simulink model "Improved_Final_Model"  (R2022a)
settings: Solver=FixedStepAuto  StartTime=0.0  StopTime=10.0  FixedStep=1e-3  RelTol=1e-3  EnableMultiTasking=on
undefined symbols (not defined in the file): a, A0, A1, b, c, D0, D1, D10, D11, D12, D13, D2, D3, D5, D6, D8, D9, PTA0, PTA1, PTA2, PTB2, PTB3, PTB9, PTC16, PTC17, PTC2, PTC4, PTD0, PTD1, PTD2, PTD3
libraries: frdmk64flib x17, simulink x2, hdlsllib x1
settings Model: ExtModeTrigDuration=5  Creator=pauls  LastModifiedBy=pauls
settings OptimizationCC: EnhancedBackFolding=on  PassReuseOutputArgsAs=Individual arguments  ZeroExternalMemoryAtStartup=off  ZeroInternalMemoryAtStartup=off  MaxStackSize=64  OptimizeBlockOrder=speed  DifferentSizesBufferReuse=on  OptimizationCustomize=off  EfficientTunableParamExpr=on
settings DebuggingCC: ParameterTunabilityLossMsg=error
settings HardwareCC: ProdBitPerPointer=32  ProdBitPerSizeT=32  ProdBitPerPtrDiffT=32  ProdLargestAtomicInteger=Long  ProdLargestAtomicFloat=Double  ProdWordSize=32  ProdHWDeviceType=ARM Compatible->ARM Cortex
settings SFSimCC: MATLABDynamicMemAlloc=off
settings RTWCC: SystemTargetFile=ert.tlc  HardwareBoard=NXP FRDM-K64F  TLCOptions="-aInlineSetEventsForThisBaseRateFcn=TLC_FALSE -aSuppressMultiTaskScheduler=TLC_FALSE  -aRateBasedStepFcn=0"  TemplateMakefile=ert_default_tmf  Toolchain=GNU Tools for ARM Embedded Processors
settings CodeAppCC: ForceParamTrailComments=on  IgnoreCustomStorageClasses=off  OperatorAnnotations=on  SimulinkDataObjDesc=on  SFDataObjDesc=on  InsertBlockDesc=on
settings ERTTargetCC: ExtModeTransport=4  ExtModeMexFile=sendToCommService

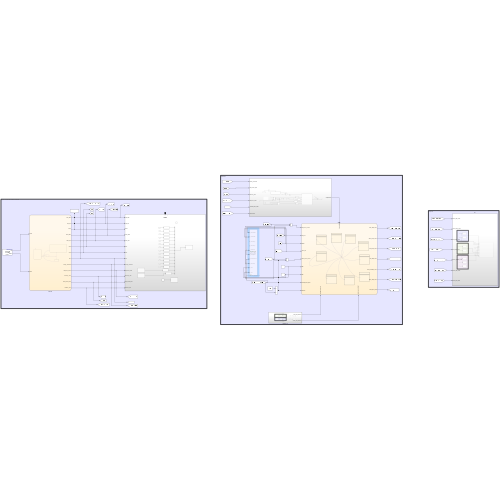
[thumbnail: Simulink's stored preview of the top-level diagram]
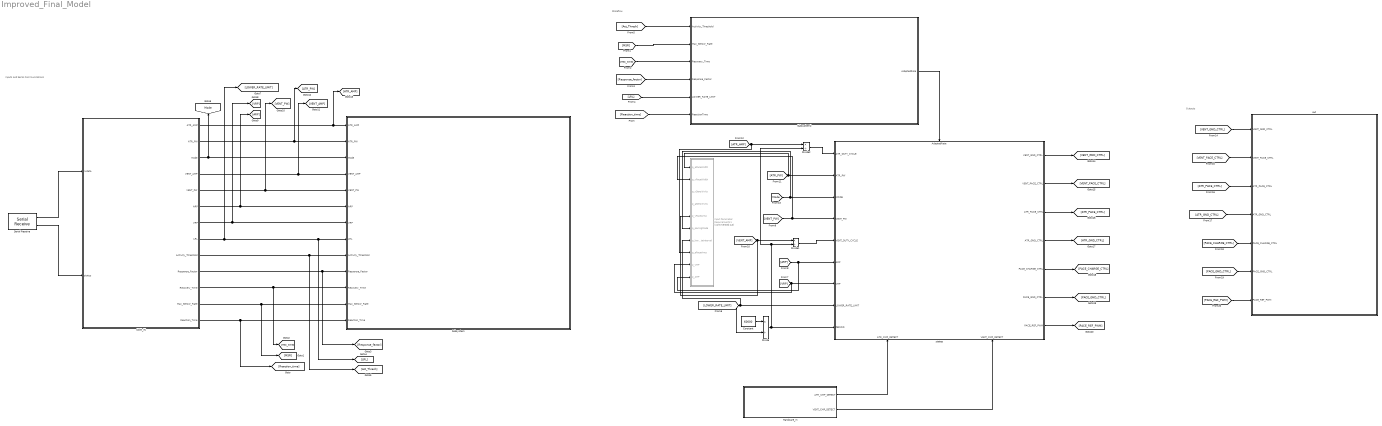
== system Improved_Final_Model ==
  note: Outputs
  note: Stateflow
  note: Inputs and Serial Communications
  " states  " : Stateflow chart  TreatAsAtomicUnit=on
      settings: PortSchema="{\"entries\":[{\"content\":{\"sides\":[{\"content\":{\"connectorIds\":[\"In7\",\"In8\",\"In2\",\"In5\",\"In6\",\"In11\",\"In10\",\"In12\",\"In9\"]},\"type\":\"ConnectorPlacement.EquallySpacedRectSide\",\"uuid\":\"01118a3a-35ab-415d-a4dc-7a9e5022dc58\"},{\"content\":{\"connectorIds\":[\"Out1\",\"Out2\",\"Out3\",\"Out4\",\"Out5\",\"Out6\",\"Out7\"],\"side\":\"RIGHT\"},\"type\":\"ConnectorPlacement.EquallySpacedRectSide\",\"uuid\":\"d119b6db-c579-45b6-8580-2a3960ab3129\"},{\"content\":{\"connectorIds\":[\"In1\"],\"side\":\"TOP\"},\"type\":\"ConnectorPlacement.EquallySpacedRectSide\",\"uuid\":\"18fa5379-1691-4053-811b-8d647a346445\"},{\"content\":{\"connectorIds\":[\"In3\",\"In4\"],\"side\":\"BOTTOM\"},\"type\":\"ConnectorPlacement.EquallySpacedRectSide\",\"uuid\":\"c19ca9f7-b829-4e11-b03e-3e9d42b35795\"}]},\"type\":\"ConnectorPlacement.EquallySpacedConnector\",\"uuid\":\"6e6fa963-33ea-4c14-97b4-73e5587667a9\"}],\"packageUris\":[\"http://schema.mathworks.com/mf0/Connector/R2020b\"],\"version\":\"1.0\"}"
  COM_IN : Stateflow chart  TreatAsAtomicUnit=on
      settings: PortSchema="{\"entries\":[{\"content\":{\"sides\":[{\"content\":{\"connectorIds\":[\"In1\",\"In2\"]},\"type\":\"ConnectorPlacement.EquallySpacedRectSide\",\"uuid\":\"47dbc3b1-cfb0-4419-87af-22cc7bee4e7f\"},{\"content\":{\"connectorIds\":[\"Out2\",\"Out1\",\"Out3\",\"Out4\",\"Out5\",\"Out6\",\"Out7\",\"Out8\",\"Out9\",\"Out10\",\"Out11\",\"Out12\",\"Out13\"],\"side\":\"RIGHT\"},\"type\":\"ConnectorPlacement.EquallySpacedRectSide\",\"uuid\":\"7e5976fa-7974-49bc-a061-2d3361778a3d\"},{\"content\":{\"connectorIds\":[],\"side\":\"TOP\"},\"type\":\"ConnectorPlacement.EquallySpacedRectSide\",\"uuid\":\"f4969c99-fcc1-4334-9f12-327b19c61b40\"}]},\"type\":\"ConnectorPlacement.EquallySpacedConnector\",\"uuid\":\"ac43404f-f257-440c-be82-ec9e7dd20d0c\"}],\"packageUris\":[\"http://schema.mathworks.com/mf0/Connector/R2020b\"],\"version\":\"1.0\"}"
  Constant : Constant  Value=60000
  Divide : Product  Inputs=*/
  Divide1 : Product  Inputs=*/
  Divide2 : Product  Inputs=*/
  Hardware_in : Subsystem
  Input Parameter Requirements1 : Requirements Table  Commented=on  TreatAsAtomicUnit=on
  Serial Receive : frdmk64flib/Serial Receive  SCIModule=0  Baudrate=uint32(9600)  Parity=None  StopBits=1  HardwareFlowControl=None  ByteOrder=LittleEndian  DataType=uint8  DataLength=15  BlockingMode=off  OutputStatus=on  SampleTime=-1
  Subsystem : Subsystem
  Subsystem2 : Subsystem
  "out " : Subsystem
  tag scope: Mode=global
  wires:
  Serial Receive/1 -> COM_IN/1(rxdata)
  Serial Receive/2 -> COM_IN/2(status)
  COM_IN/1(ATR_PW) -> [ATR_PW], Subsystem/2(ATR_PW)
  COM_IN/2(ATR_AMP) -> [ATR_AMP], Subsystem/1(ATR_AMP)
  COM_IN/3(Mode) -> Subsystem/3(Mode), [Mode]
  COM_IN/4(VENT_AMP) -> [VENT_AMP], Subsystem/4(VENT_AMP)
  COM_IN/5(VENT_PW) -> [VENT_PW], Subsystem/5(VENT_PW)
  COM_IN/6(ARP) -> [ARP], Subsystem/6(ARP)
  COM_IN/7(VRP) -> [VRP], Subsystem/7(VRP)
  COM_IN/8(LRL) -> [LOWER_RATE_LIMIT], [LRL], Subsystem/8(LRL)
  COM_IN/9(Activity_Threshold) -> [Act_Thresh], Subsystem/9(Activity_Threshold)
  COM_IN/10(Response_Factor) -> [Response_factor], Subsystem/10(Response_Factor)
  COM_IN/11(Recovery_Time) -> [Rec_time], Subsystem/11(Recovery_Time)
  COM_IN/12(Max_Sensor_Rate) -> [MSR], Subsystem/12(Max_Sensor_Rate)
  COM_IN/13(Reaction_Time) -> Subsystem/13(Reaction_Time), [Reaction_time]
  Hardware_in/1(ATR_CMP_DETECT) -> " states  "/3(ATR_CMP_DETECT)
  Hardware_in/2(VENT_CMP_DETECT) -> " states  "/4(VENT_CMP_DETECT)
  Divide/1 -> Divide1/2, Divide2/2, " states  "/9(PERIOD)
  Constant/1 -> Divide/1
  [Rec_time] -> Subsystem2/3(Recovery_Time)
  [Response_factor] -> Subsystem2/4(Response_Factor)
  [LRL] -> Subsystem2/5(LOWER_RATE_LIMIT)
  [Reaction_time] -> Subsystem2/6(ReactionTime)
  [Act_Thresh] -> Subsystem2/1(Activity_Threshold)
  [MSR] -> Subsystem2/2(Max_Sensor_Rate)
  Subsystem2/1(AdaptedRate) -> " states  "/1(AdaptedRate)
  [LOWER_RATE_LIMIT] -> Input Parameter Requirements1/7(p_lowrateInterval), " states  "/12(LOWER_RATE_LIMIT), Divide/2
  [VRP] -> Input Parameter Requirements1/9(p_VRP), " states  "/10(VRP)
  [ARP] -> Input Parameter Requirements1/10(p_ARP), " states  "/11(ARP)
  [ATR_PW] -> Input Parameter Requirements1/1(p_aPaceWidth), " states  "/8(ATR_PW)
  [VENT_AMP] -> Input Parameter Requirements1/5(p_vPaceAmp), Divide1/1
  [VENT_PW] -> Input Parameter Requirements1/2(p_vPaceWidth), " states  "/5(VENT_PW)
  [ATR_AMP] -> Input Parameter Requirements1/8(p_aPaceAmp), Divide2/1
  [Mode] -> Input Parameter Requirements1/6(p_pacingMode), " states  "/2(MODE)
  " states  "/1(VENT_GND_CTRL) -> [VENT_GND_CTRL]
  " states  "/2(VENT_PACE_CTRL) -> [VENT_PACE_CTRL]
  " states  "/3(ATR_PACE_CTRL) -> [ATR_PACE_CTRL]
  " states  "/4(ATR_GND_CTRL) -> [ATR_GND_CTRL]
  " states  "/5(PACE_CHARGE_CTRL) -> [PACE_CHARGE_CTRL]
  " states  "/6(PACE_GND_CTRL) -> [PACE_GND_CTRL]
  " states  "/7(PACE_REF_PWM) -> [PACE_REF_PWM]
  [VENT_GND_CTRL] -> "out "/1(VENT_GND_CTRL)
  [VENT_PACE_CTRL] -> "out "/2(VENT_PACE_CTRL)
  [ATR_PACE_CTRL] -> "out "/3(ATR_PACE_CTRL)
  [ATR_GND_CTRL] -> "out "/4(ATR_GND_CTRL)
  [PACE_CHARGE_CTRL] -> "out "/5(PACE_CHARGE_CTRL)
  [PACE_GND_CTRL] -> "out "/6(PACE_GND_CTRL)
  [PACE_REF_PWM] -> "out "/7(PACE_REF_PWM)
  Divide1/1 -> " states  "/6(VENT_DUTY_CYCLE)
  Divide2/1 -> " states  "/7(ATR_DUTY_CYCLE)

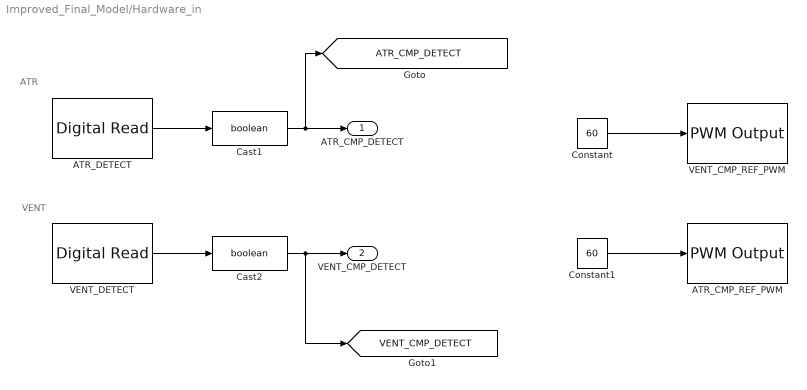
== system Improved_Final_Model/Hardware_in ==
  note: VENT
  note: ATR
  ATR_CMP_REF_PWM : frdmk64flib/PWM Output  Whichpin=PTC2 (D6)  InitialFrequency=2000  InitialDutyCycle=52
  ATR_DETECT : frdmk64flib/Digital Read  Whichpin=PTC16 (D0)  SampleTime=-1
  Cast1 : DataTypeConversion  OutDataTypeStr=boolean  SaturateOnIntegerOverflow=off  RndMeth=Floor
  Cast2 : DataTypeConversion  OutDataTypeStr=boolean  SaturateOnIntegerOverflow=off  RndMeth=Floor
  Constant : Constant  Value=60
  Constant1 : Constant  Value=60
  VENT_CMP_REF_PWM : frdmk64flib/PWM Output  Whichpin=PTA1 (D3)  InitialFrequency=2000  InitialDutyCycle=52
  VENT_DETECT : frdmk64flib/Digital Read  Whichpin=PTC17 (D1)  SampleTime=-1
  ATR_CMP_DETECT : Outport
  VENT_CMP_DETECT : Outport  Port=2
  tag scope: ATR_CMP_DETECT=global, VENT_CMP_DETECT=global
  wires:
  Cast1/1 -> ATR_CMP_DETECT/1, [ATR_CMP_DETECT]
  ATR_DETECT/1 -> Cast1/1
  VENT_DETECT/1 -> Cast2/1
  Cast2/1 -> [VENT_CMP_DETECT], VENT_CMP_DETECT/1
  Constant/1 -> VENT_CMP_REF_PWM/1
  Constant1/1 -> ATR_CMP_REF_PWM/1

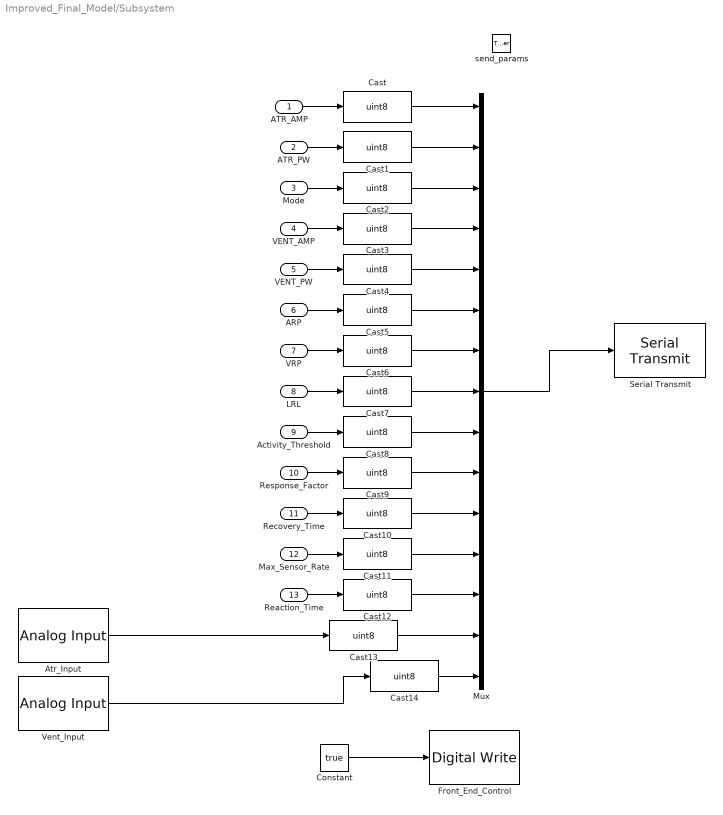
== system Improved_Final_Model/Subsystem ==
  ATR_AMP : Inport
  ATR_PW : Inport  Port=2
  Mode : Inport  Port=3
  VENT_AMP : Inport  Port=4
  VENT_PW : Inport  Port=5
  ARP : Inport  Port=6
  VRP : Inport  Port=7
  LRL : Inport  Port=8
  Activity_Threshold : Inport  Port=9
  Response_Factor : Inport  Port=10
  Recovery_Time : Inport  Port=11
  Max_Sensor_Rate : Inport  Port=12
  Reaction_Time : Inport  Port=13
  send_params : TriggerPort  TriggerType=function-call  IsSimulinkFunction=on  FunctionName=send_Test  VariantControl=(inherit)
  Atr_Input : frdmk64flib/Analog Input  Whichpin=PTB2 (A0)  SampleTime=-1
  Cast{,1..14} (15 alike) : DataTypeConversion  OutDataTypeStr=uint8  SaturateOnIntegerOverflow=off  RndMeth=Floor
  Constant : Constant  Value=true
  Front_End_Control : frdmk64flib/Digital Write  Whichpin=PTD1 (D13)
  Mux : Mux  Inputs=15
  Serial Transmit : frdmk64flib/Serial Transmit  SCIModule=0  Baudrate=uint32(9600)  Parity=None  StopBits=1  HardwareFlowControl=None  ByteOrder=LittleEndian  BlockingMode=on  OutputStatus=off
  Vent_Input : frdmk64flib/Analog Input  Whichpin=PTB3 (A1)  SampleTime=-1
  wires:
  ATR_AMP/1 -> Cast/1
  Mux/1 -> Serial Transmit/1
  ATR_PW/1 -> Cast1/1
  Cast1/1 -> Mux/2
  Cast/1 -> Mux/1
  Mode/1 -> Cast2/1
  Cast2/1 -> Mux/3
  VENT_AMP/1 -> Cast3/1
  VENT_PW/1 -> Cast4/1
  ARP/1 -> Cast5/1
  VRP/1 -> Cast6/1
  LRL/1 -> Cast7/1
  Cast3/1 -> Mux/4
  Cast4/1 -> Mux/5
  Cast5/1 -> Mux/6
  Cast6/1 -> Mux/7
  Cast7/1 -> Mux/8
  Cast8/1 -> Mux/9
  Cast12/1 -> Mux/13
  Cast11/1 -> Mux/12
  Cast9/1 -> Mux/10
  Cast10/1 -> Mux/11
  Response_Factor/1 -> Cast9/1
  Activity_Threshold/1 -> Cast8/1
  Recovery_Time/1 -> Cast10/1
  Reaction_Time/1 -> Cast12/1
  Max_Sensor_Rate/1 -> Cast11/1
  Constant/1 -> Front_End_Control/1
  Atr_Input/1 -> Cast13/1
  Vent_Input/1 -> Cast14/1
  Cast13/1 -> Mux/14
  Cast14/1 -> Mux/15

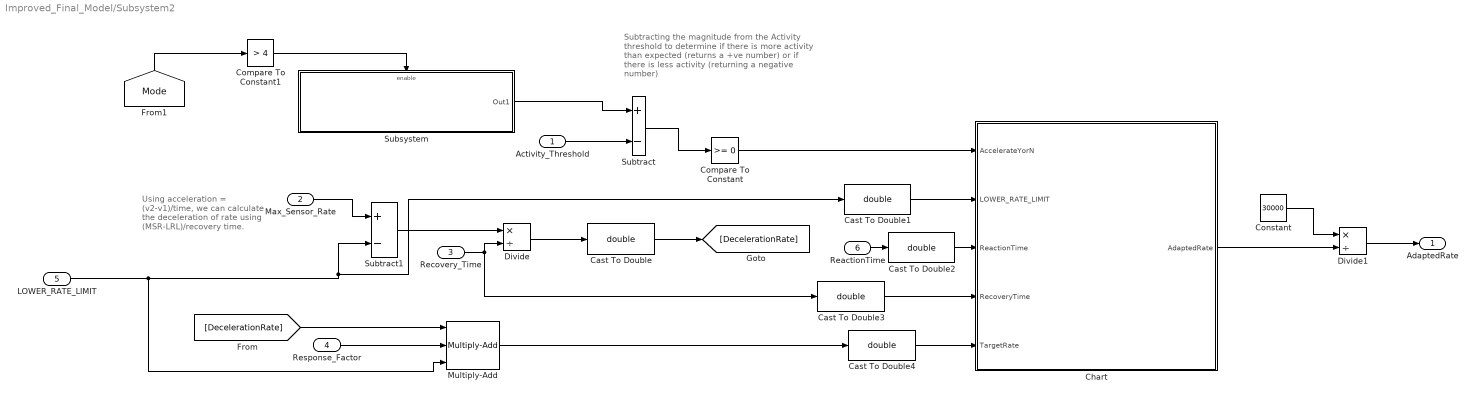
== system Improved_Final_Model/Subsystem2 ==
  note: Using acceleration = (v2-v1)/time, we can calculate the deceleration of rate using
      | (MSR-LRL)/recovery time.
  note: Subtracting the magnitude from the Activity threshold to determine if there is more activity than expected (returns a +ve number) or if there is less activity (returning a negative number)
  Activity_Threshold : Inport
  Max_Sensor_Rate : Inport  Port=2
  Recovery_Time : Inport  Port=3
  Response_Factor : Inport  Port=4
  LOWER_RATE_LIMIT : Inport  Port=5
  ReactionTime : Inport  Port=6
  Cast To Double{,1..4} (5 alike) : DataTypeConversion  OutDataTypeStr=double  SaturateOnIntegerOverflow=off  RndMeth=Floor
  Chart : Stateflow chart  TreatAsAtomicUnit=on
      settings: PortSchema="{\"entries\":[{\"content\":{\"sides\":[{\"content\":{\"connectorIds\":[\"In2\",\"In1\",\"In3\",\"In4\",\"In5\"]},\"type\":\"ConnectorPlacement.EquallySpacedRectSide\",\"uuid\":\"6eaaa5c3-a67e-4334-8771-4d714dd3c2aa\"},{\"content\":{\"connectorIds\":[\"Out1\"],\"side\":\"RIGHT\"},\"type\":\"ConnectorPlacement.EquallySpacedRectSide\",\"uuid\":\"be5e1652-7b89-433f-97fe-a51584ee4ad6\"},{\"content\":{\"connectorIds\":[],\"side\":\"TOP\"},\"type\":\"ConnectorPlacement.EquallySpacedRectSide\",\"uuid\":\"88923a53-eca7-4a95-abe6-229d007878e0\"}]},\"type\":\"ConnectorPlacement.EquallySpacedConnector\",\"uuid\":\"0db105c6-87da-444f-9a1d-26abcd68563f\"}],\"packageUris\":[\"http://schema.mathworks.com/mf0/Connector/R2020b\"],\"version\":\"1.0\"}"
  Compare To Constant : simulink/Logic and Bit Operations/Compare To Constant  relop=>=  const=0  OutDataTypeStr=boolean
  Compare To Constant1 : simulink/Logic and Bit Operations/Compare To Constant  relop=>  const=4  OutDataTypeStr=boolean
  Constant : Constant  Value=30000
  Divide : Product  Inputs=*/
  Divide1 : Product  Inputs=*/
  Multiply-Add : hdlsllib/HDL Operations/Multiply-Add  Function=c+(a.*b)  datatype=Inherit: Inherit via internal rule  DoSatur=off  FMA=off
      settings: SourceProductBaseCode=SL
  Subsystem : Subsystem
  Subtract : Sum  Inputs=+-
  Subtract1 : Sum  Inputs=+-
  AdaptedRate : Outport
  wires:
  Divide1/1 -> AdaptedRate/1
  Response_Factor/1 -> Multiply-Add/2
  Cast To Double2/1 -> Chart/3(ReactionTime)
  Cast To Double4/1 -> Chart/5(TargetRate)
  ReactionTime/1 -> Cast To Double2/1
  Cast To Double1/1 -> Chart/1(LOWER_RATE_LIMIT)
  [DecelerationRate] -> Multiply-Add/1
  Constant/1 -> Divide1/1
  Subtract1/1 -> Divide/1
  Cast To Double3/1 -> Chart/4(RecoveryTime)
  Chart/1(AdaptedRate) -> Divide1/2
  Recovery_Time/1 -> Cast To Double3/1, Divide/2
  LOWER_RATE_LIMIT/1 -> Multiply-Add/3, Subtract1/2, Cast To Double1/1
  Cast To Double/1 -> [DecelerationRate]
  Compare To Constant/1 -> Chart/2(AccelerateYorN)
  Divide/1 -> Cast To Double/1
  Max_Sensor_Rate/1 -> Subtract1/1
  Activity_Threshold/1 -> Subtract/2
  Subtract/1 -> Compare To Constant/1
  Multiply-Add/1 -> Cast To Double4/1
  Subsystem/1(Out1) -> Subtract/1
  [Mode] -> Compare To Constant1/1
  Compare To Constant1/1 -> Subsystem/Enable

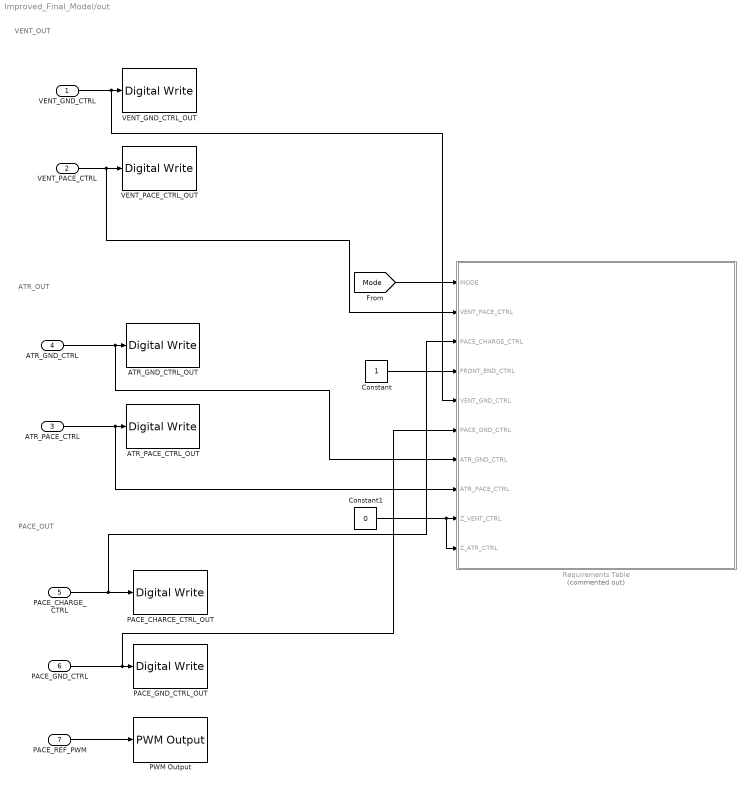
== system Improved_Final_Model/out  ==
  note: PACE_OUT
  note: ATR_OUT
  note: VENT_OUT
  VENT_GND_CTRL : Inport
  VENT_PACE_CTRL : Inport  Port=2
  ATR_PACE_CTRL : Inport  Port=3
  ATR_GND_CTRL : Inport  Port=4
  PACE_CHARGE_CTRL : Inport  Port=5
  PACE_GND_CTRL : Inport  Port=6
  PACE_REF_PWM : Inport  Port=7
  ATR_GND_CTRL_OUT : frdmk64flib/Digital Write  Whichpin=PTD2 (D11)
  ATR_PACE_CTRL_OUT : frdmk64flib/Digital Write  Whichpin=PTA0 (D8)
  Constant : Constant
  Constant1 : Constant  Value=0
  PACE_CHARCE_CTRL_OUT : frdmk64flib/Digital Write  Whichpin=PTB9 (D2)
  PACE_GND_CTRL_OUT : frdmk64flib/Digital Write  Whichpin=PTD0 (D10)
  PWM Output : frdmk64flib/PWM Output  Whichpin=PTA2 (D5)  InitialFrequency=2000  InitialDutyCycle=100
  Requirements Table : Requirements Table  Commented=on  TreatAsAtomicUnit=on
  VENT_GND_CTRL_OUT : frdmk64flib/Digital Write  Whichpin=PTD3 (D12)
  VENT_PACE_CTRL_OUT : frdmk64flib/Digital Write  Whichpin=PTC4 (D9)
  wires:
  VENT_GND_CTRL/1 -> Requirements Table/5(VENT_GND_CTRL), VENT_GND_CTRL_OUT/1
  VENT_PACE_CTRL/1 -> Requirements Table/2(VENT_PACE_CTRL), VENT_PACE_CTRL_OUT/1
  ATR_GND_CTRL/1 -> Requirements Table/7(ATR_GND_CTRL), ATR_GND_CTRL_OUT/1
  ATR_PACE_CTRL/1 -> Requirements Table/8(ATR_PACE_CTRL), ATR_PACE_CTRL_OUT/1
  PACE_CHARGE_CTRL/1 -> Requirements Table/3(PACE_CHARGE_CTRL), PACE_CHARCE_CTRL_OUT/1
  PACE_REF_PWM/1 -> PWM Output/1
  PACE_GND_CTRL/1 -> Requirements Table/6(PACE_GND_CTRL), PACE_GND_CTRL_OUT/1
  [Mode] -> Requirements Table/1(MODE)
  Constant/1 -> Requirements Table/4(FRONT_END_CTRL)
  Constant1/1 -> Requirements Table/10(Z_ATR_CTRL), Requirements Table/9(Z_VENT_CTRL)

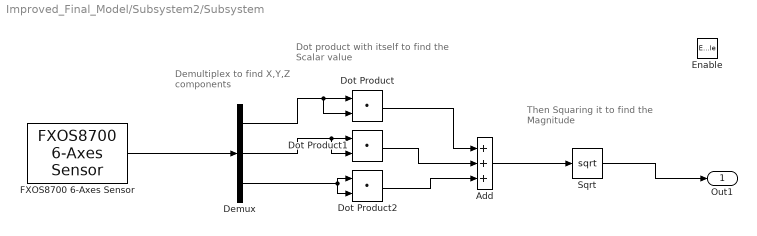
== system Improved_Final_Model/Subsystem2/Subsystem ==
  note: Demultiplex to find
      | X,Y,Z components
  note: Dot product with itself to find the
      | Scalar value
  note: Then Squaring it to find the Magnitude
  Enable : EnablePort
  Add : Sum  Inputs=+++
  Demux : Demux  Outputs=3
  Dot Product : DotProduct  OutDataTypeStr=Inherit: Inherit via internal rule
  Dot Product1 : DotProduct  OutDataTypeStr=Inherit: Inherit via internal rule
  Dot Product2 : DotProduct  OutDataTypeStr=Inherit: Inherit via internal rule
  FXOS8700 6-Axes Sensor : frdmk64flib/FXOS8700 6-Axes Sensor  Activesensor=Accelerometer only  ODR=800Hz  HybridODR=400Hz  Accelfullrange=-4g to +4g  SampleTime=-1
  Sqrt : Sqrt
  Out1 : Outport
  wires:
  Demux/3 -> Dot Product2/2, Dot Product2/1
  Demux/2 -> Dot Product1/2, Dot Product1/1
  Demux/1 -> Dot Product/2, Dot Product/1
  FXOS8700 6-Axes Sensor/1 -> Demux/1
  Dot Product2/1 -> Add/3
  Dot Product/1 -> Add/1
  Add/1 -> Sqrt/1
  Dot Product1/1 -> Add/2
  Sqrt/1 -> Out1/1

== stateflow chart Improved_Final_Model/ states   ==
  state Default [group]
    state CharingC23
      during:
      %Begin Charging C22 Capacitor
      VENT_PACE_CTRL = LOW;
      PACE_REF_PWM = (VENT_DUTY_CYCLE/5)*100;
      PACE_CHARGE_CTRL = HIGH;
      %Begin Discharging C21 Blocking Capacitor
      PACE_GND_CTRL = HIGH;
      VENT_PACE_CTRL = LOW;
      VENT_GND_CTRL = HIGH;
    state Discharge
      during:
      %Discharge C22 into Ventricle (Vent Pacing)
      %Begin Charging Blocking Capacitor
      PACE_CHARGE_CTRL = LOW;
      PACE_GND_CTRL = HIGH;
      VENT_GND_CTRL = LOW;
      VENT_PACE_CTRL  = HIGH;
    Default.CharingC23 -> Default.Discharge : after(PERIOD-VENT_PW, msec)
    Default.Discharge -> Default.CharingC23 : after(VENT_PW, msec)
  state AOO [group]
    state CharingC22
      %Capacitor charing state
      ATR_PACE_CTRL = LOW
      PACE_REF_PWM = (ATR_DUTY_CYCLE/5)*100
      PACE_CHARGE_CTRL = HIGH
      %Discharge capacitor
      PACE_GND_CTRL = HIGH
      ATR_PACE_CTRL = LOW
      ATR_GND_CTRL = HIGH
    state AVPacing
      %step 2
      PACE_CHARGE_CTRL = LOW
      PACE_GND_CTRL = HIGH
      ATR_PACE_CTRL = HIGH
      ATR_GND_CTRL = LOW
    AOO.CharingC22 -> AOO.AVPacing : after(PERIOD-ATR_PW, msec)
    AOO.AVPacing -> AOO.CharingC22 : after(ATR_PW, msec)
  state VVIR [group]
    state DISCHARGING
      during:
      %Step 1:
      %Discharge C22 into Ventricle (Vent Pacing)
      %Begin Charging Blocking Capacitor
      PACE_CHARGE_CTRL = LOW
      PACE_GND_CTRL = HIGH
      VENT_GND_CTRL = LOW
      VENT_PACE_CTRL  = HIGH
    state CHARGING
      during:
      %Begin Charging C22 Capacitor
      VENT_PACE_CTRL = LOW;
      PACE_REF_PWM = (VENT_DUTY_CYCLE/5)*100;
      PACE_CHARGE_CTRL = HIGH;
      %Begin Discharging C21 Blocking Capacitor
      PACE_GND_CTRL = HIGH;
      VENT_PACE_CTRL = LOW;
      VENT_GND_CTRL = HIGH;
    state PROXY
      during:
      PACE_GND_CTRL = HIGH;
      VENT_PACE_CTRL = LOW;
      VENT_GND_CTRL = HIGH;
    CHARGING -> VVIR.DISCHARGING : after(AdaptedRate-VENT_PW-VRP, msec)
    VVIR.DISCHARGING -> (junction 195) [order 2] : after(LOWER_RATE_LIMIT,msec)
    (junction 195) -> PROXY : [VENT_CMP_DETECT==HIGH]
    VVIR.DISCHARGING -> PROXY [order 1] : after(VENT_PW, msec)
    PROXY -> CHARGING : after(VRP, msec)
  state VOO [group]
    state CharingC23
      during:
      %Begin Charging C22 Capacitor
      VENT_PACE_CTRL = LOW;
      PACE_REF_PWM = (VENT_DUTY_CYCLE/PERIOD);
      PACE_CHARGE_CTRL = HIGH;
      %Begin Discharging C21 Blocking Capacitor
      PACE_GND_CTRL = HIGH;
      VENT_PACE_CTRL = LOW;
      VENT_GND_CTRL = HIGH;
    state Discharge
      during:
      %Discharge C22 into Ventricle (Vent Pacing)
      %Begin Charging Blocking Capacitor
      PACE_CHARGE_CTRL = LOW;
      PACE_GND_CTRL = HIGH;
      VENT_GND_CTRL = LOW;
      VENT_PACE_CTRL  = HIGH;
    VOO.CharingC23 -> VOO.Discharge : after(PERIOD-VENT_PW, msec)
    VOO.Discharge -> VOO.CharingC23 : after(VENT_PW, msec)
  state AAIR [group]
    state DISCHARGING
      during:
      %Discharge C22 into Atrium (Atrial Pacing)
      %Begin Charging Blocking Capacitor
      PACE_CHARGE_CTRL = LOW
      PACE_GND_CTRL = HIGH
      ATR_PACE_CTRL = HIGH
      ATR_GND_CTRL = LOW
    state CharingC23
      during:
      %Begin Charging C22 Capacitor
      ATR_PACE_CTRL = LOW
      PACE_REF_PWM = (ATR_DUTY_CYCLE/5)*100
      PACE_CHARGE_CTRL = HIGH
      %Begin Discharging C21 Blocking Capacitor
      PACE_GND_CTRL = HIGH
      ATR_PACE_CTRL = LOW
      ATR_GND_CTRL = HIGH
    state Proxy
      during:
      PACE_GND_CTRL = HIGH
      ATR_PACE_CTRL = LOW
      ATR_GND_CTRL = HIGH
    AAIR.CharingC23 -> AAIR.DISCHARGING : after(AdaptedRate-ATR_PW-ARP, msec)
    AAIR.DISCHARGING -> (junction 178) [order 2] : after(LOWER_RATE_LIMIT,msec)
    (junction 178) -> Proxy : [ATR_CMP_DETECT==HIGH]
    AAIR.DISCHARGING -> Proxy [order 1] : after(ATR_PW, msec)
    Proxy -> AAIR.CharingC23 : after(ARP, msec)
  state VVI [group]
    state CharingC23
      during:
      %Begin Charging C22 Capacitor
      VENT_PACE_CTRL = LOW;
      PACE_REF_PWM = (VENT_DUTY_CYCLE/5)*100;
      PACE_CHARGE_CTRL = HIGH;
      %Begin Discharging C21 Blocking Capacitor
      PACE_GND_CTRL = HIGH;
      VENT_PACE_CTRL = LOW;
      VENT_GND_CTRL = HIGH;
    state Discharge
      during:
      %Discharge C22 into Ventricle (Vent Pacing)
      %Begin Charging Blocking Capacitor
      PACE_CHARGE_CTRL = LOW
      PACE_GND_CTRL = HIGH
      VENT_GND_CTRL = LOW
      VENT_PACE_CTRL  = HIGH
    state Inhibit
      PACE_GND_CTRL = HIGH
      VENT_PACE_CTRL = LOW
      VENT_GND_CTRL = HIGH
    VVI.CharingC23 -> VVI.Discharge [order 1] : after(PERIOD-VENT_PW, msec)[VENT_CMP_DETECT == LOW]
    VVI.CharingC23 -> VVI.Inhibit [order 2] : after(LOWER_RATE_LIMIT, msec)[VENT_CMP_DETECT == HIGH]
    VVI.Inhibit -> VVI.CharingC23 : after(VRP,msec)
    VVI.Discharge -> VVI.Inhibit : after(VENT_PW, msec)
  state AAI [group]
    state AVPacing
      %step 2
      PACE_CHARGE_CTRL = LOW
      PACE_GND_CTRL = HIGH
      ATR_PACE_CTRL = HIGH
      ATR_GND_CTRL = LOW
    state CharingC22
      %Capacitor charing state
      ATR_PACE_CTRL = LOW
      PACE_REF_PWM = (ATR_DUTY_CYCLE/5)*100
      PACE_CHARGE_CTRL = HIGH
      %Discharge capacitor
      PACE_GND_CTRL = HIGH
      ATR_PACE_CTRL = LOW
      ATR_GND_CTRL = HIGH
    state Inhibit
      %Through Trial and error found that discharging
      %again will fix the pacing during AAI
      PACE_GND_CTRL = HIGH
      ATR_PACE_CTRL = LOW
      ATR_GND_CTRL = LOW
    AAI.CharingC22 -> AAI.AVPacing [order 2] : after(PERIOD-ATR_PW, msec)
    AAI.CharingC22 -> AAI.Inhibit [order 1] : after(LOWER_RATE_LIMIT,msec)[ATR_CMP_DETECT == HIGH]
    AAI.AVPacing -> AAI.Inhibit : after(ATR_PW, msec)
    AAI.Inhibit -> AAI.CharingC22 : after(ARP,msec)
  state VOOR [group]
    state CharingC23
      during:
      %Begin Charging C22 Capacitor
      VENT_PACE_CTRL = LOW
      PACE_REF_PWM = (VENT_DUTY_CYCLE/5)*100
      PACE_CHARGE_CTRL = HIGH
      %Begin Discharging C21 Blocking Capacitor
      PACE_GND_CTRL = HIGH
      VENT_PACE_CTRL = LOW
      VENT_GND_CTRL = HIGH
    state AVPacing1
      during:
      %Discharge C22 into Ventricle (Vent Pacing)
      %Begin Charging Blocking Capacitor
      PACE_CHARGE_CTRL = LOW
      PACE_GND_CTRL = HIGH
      VENT_GND_CTRL = LOW
      VENT_PACE_CTRL  = HIGH
    VOOR.CharingC23 -> AVPacing1 : after(AdaptedRate-ATR_PW, msec)
    AVPacing1 -> VOOR.CharingC23 : after(ATR_PW, msec)
  state AOOR [group]
    state CharingC23
      during:
      %Begin Charging C22 Capacitor
      ATR_PACE_CTRL = LOW
      PACE_REF_PWM = (ATR_DUTY_CYCLE/5)*100
      PACE_CHARGE_CTRL = HIGH
      %Begin Discharging C21 Blocking Capacitor
      PACE_GND_CTRL = HIGH
      ATR_PACE_CTRL = LOW
      ATR_GND_CTRL = HIGH
    state Discharge
      during:
      %Discharge C22 into Atrium (AtrialPacing)
      %Begin Charging C21 Blocking Capacitor
      PACE_CHARGE_CTRL = LOW
      PACE_GND_CTRL = HIGH
      ATR_PACE_CTRL = HIGH
      ATR_GND_CTRL = LOW
    AOOR.CharingC23 -> AOOR.Discharge : after(AdaptedRate-ATR_PW, msec)
    AOOR.Discharge -> AOOR.CharingC23 : after(ATR_PW, msec)
  (junction 211) -> CHARGING [order 8] : [MODE==8]
  (junction 211) -> Default.CharingC23 [order 9]
  (default) -> (junction 211)
  (junction 211) -> VOOR.CharingC23 [order 6] : [MODE == 6]
  (junction 211) -> AAIR.CharingC23 [order 7] : [MODE == 7]
  (junction 211) -> AOOR.CharingC23 [order 5] : [MODE ==5]
  (junction 211) -> VVI.CharingC23 [order 3] : [MODE ==3]
  (junction 211) -> AAI.CharingC22 [order 4] : [MODE == 4]
  (junction 211) -> AOO.CharingC22 [order 1] : [MODE ==1]
  (junction 211) -> VOO.CharingC23 [order 2] : [MODE ==2]
  data: AdaptedRate input; MODE input; ATR_CMP_DETECT input; VENT_CMP_DETECT input; VENT_GND_CTRL output; VENT_PACE_CTRL output; ATR_PACE_CTRL output; VENT_PW input; VENT_DUTY_CYCLE input; HIGH local =true; LOW local =false; ATR_GND_CTRL output; PACE_CHARGE_CTRL output; PACE_GND_CTRL output; PACE_REF_PWM output; ATR_DUTY_CYCLE input; ATR_PW input; PERIOD input; VRP input; ARP input; LOWER_RATE_LIMIT input

== stateflow chart Improved_Final_Model/out /Requirements Table ==
  (default) -> (junction 1073745709)
  (junction 1073745709) -> (junction 1073745710) : {
      | % SF_REQ_REV_07
      | }
  (junction 1073745710) -> (junction 1073745712) : {
      | % HEADER_ASSIGNMENTS
      |
      | }
  (junction 1073745712) -> (junction 1073745714) : {
      | % START_A_4
      | }
  (junction 1073745714) -> (junction 1073745716) : {
      | }
  (junction 1073745716) -> (junction 1073745718)
  (junction 1073745718) -> (junction 1073745720) : {
      | }
  (junction 1073745720) -> (junction 1073745722) : {
      | % END_A_4
      | }
  (junction 1073745722) -> (junction 1073745724) : {
      | % START_R_1
      | }
  (junction 1073745724) -> (junction 1073745726) : {
      | }
  (junction 1073745726) -> (junction 1073745728)
  (junction 1073745728) -> (junction 1073745730) [order 1] : [(((PACE_CHARGE_CTRL) == (true))) && ((ATR_PACE_CTRL) | VENT_PACE_CTRL ) && ((VENT_PACE_CTRL ) | ATR_PACE_CTRL)]
  (junction 1073745728) -> (junction 1073745736) [order 2]
  (junction 1073745730) -> (junction 1073745732) : {
      | reqtable_postcondition((PACE_GND_CTRL ~= PACE_GND_CTRL) && (((Z_ATR_CTRL) == (false))) && (((Z_VENT_CTRL) == (false))), 'R:1');
      |
      |
      | }
  (junction 1073745732) -> (junction 1073745734) : {
      | }
  (junction 1073745734) -> (junction 1073745736)
  (junction 1073745736) -> (junction 1073745738)
  (junction 1073745738) -> (junction 1073745740) : {
      | % END_R_1
      | }
  (junction 1073745740) -> (junction 1073745742) : {
      | % START_R_25
      | }
  (junction 1073745742) -> (junction 1073745744) : {
      | }
  (junction 1073745744) -> (junction 1073745746)
  (junction 1073745746) -> (junction 1073745748) [order 1] : [(((ATR_PACE_CTRL) == (true))) && (((VENT_PACE_CTRL ) == (true)))]
  (junction 1073745746) -> (junction 1073745754) [order 2]
  (junction 1073745748) -> (junction 1073745750) : {
      | reqtable_postcondition((PACE_GND_CTRL ~= PACE_GND_CTRL) && (((Z_ATR_CTRL) == (false))) && (((Z_VENT_CTRL) == (false))), 'R:2');
      |
      |
      | }
  (junction 1073745750) -> (junction 1073745752) : {
      | }
  (junction 1073745752) -> (junction 1073745754)
  (junction 1073745754) -> (junction 1073745756)
  (junction 1073745756) -> (junction 1073745758) : {
      | % END_R_25
      | }
  (junction 1073745758) -> (junction 1073745760) : {
      | % START_R_7
      | }
  (junction 1073745760) -> (junction 1073745762) : {
      | }
  (junction 1073745762) -> (junction 1073745764)
  (junction 1073745764) -> (junction 1073745766) [order 1] : [(((MODE) == (3)) || ((MODE) == (4)) || ((MODE) == (7)) || ((MODE) == (8)))]
  (junction 1073745764) -> (junction 1073745772) [order 2]
  (junction 1073745766) -> (junction 1073745768) : {
      | reqtable_postcondition((PACE_GND_CTRL == true) && (((ATR_GND_CTRL ) == (false))) && (((VENT_GND_CTRL ) == (false))) && (((FRONT_END_CTRL ) == (true))) && (((Z_ATR_CTRL) == (false))) && (((Z_VENT_CTRL) == (false))), 'R:3');
      |
      |
      | }
  (junction 1073745768) -> (junction 1073745770) : {
      | }
  (junction 1073745770) -> (junction 1073745772)
  (junction 1073745772) -> (junction 1073745774)
  (junction 1073745774) -> (junction 1073745776) : {
      | % END_R_7
      | }
  (junction 1073745776) -> (junction 1073745778) : {
      | % START_R_19
      | }
  (junction 1073745778) -> (junction 1073745780) : {
      | }
  (junction 1073745780) -> (junction 1073745782)
  (junction 1073745782) -> (junction 1073745784) [order 1] : [(((PACE_CHARGE_CTRL) == (true))) && (((ATR_PACE_CTRL) == (false))) && (((VENT_PACE_CTRL ) == (false)))]
  (junction 1073745782) -> (junction 1073745790) [order 2]
  (junction 1073745784) -> (junction 1073745786) : {
      | reqtable_postcondition((PACE_GND_CTRL == true) && (((ATR_GND_CTRL ) == (false))) && (((VENT_GND_CTRL ) == (false))) && (((FRONT_END_CTRL ) == (true))) && (((Z_ATR_CTRL) == (false))) && (((Z_VENT_CTRL) == (false))), 'R:4');
      |
      |
      | }
  (junction 1073745786) -> (junction 1073745788) : {
      | }
  (junction 1073745788) -> (junction 1073745790)
  (junction 1073745790) -> (junction 1073745792)
  (junction 1073745792) -> (junction 1073745794) : {
      | % END_R_19
      | }
  (junction 1073745794) -> (junction 1073745796) : {
      | % START_R_13
      | }
  (junction 1073745796) -> (junction 1073745798) : {
      | }
  (junction 1073745798) -> (junction 1073745800)
  (junction 1073745800) -> (junction 1073745802) [order 1] : [(((MODE) == (1)) || ((MODE) == (4)) || ((MODE) == (5)) || ((MODE) == (7))) && (((PACE_CHARGE_CTRL) == (false))) && (((ATR_PACE_CTRL) == (true))) && (((VENT_PACE_CTRL ) == (false)))]
  (junction 1073745800) -> (junction 1073745808) [order 2]
  (junction 1073745802) -> (junction 1073745804) : {
      | reqtable_postcondition((PACE_GND_CTRL == true) && (((ATR_GND_CTRL ) == (true))) && (((VENT_GND_CTRL ) == (false))) && (((FRONT_END_CTRL ) == (true))) && (((Z_ATR_CTRL) == (false))) && (((Z_VENT_CTRL) == (false))), 'R:5');
      |
      |
      | }
  (junction 1073745804) -> (junction 1073745806) : {
      | }
  (junction 1073745806) -> (junction 1073745808)
  (junction 1073745808) -> (junction 1073745810)
  (junction 1073745810) -> (junction 1073745812) : {
      | % END_R_13
      | }
  (junction 1073745812) -> (junction 1073745814) : {
      | % START_R_16
      | }
  (junction 1073745814) -> (junction 1073745816) : {
      | }
  (junction 1073745816) -> (junction 1073745818)
  (junction 1073745818) -> (junction 1073745820) [order 1] : [(((MODE) == (2)) || ((MODE) == (3)) || ((MODE) == (6)) || ((MODE) == (8))) && (((PACE_CHARGE_CTRL) == (false))) && (((ATR_PACE_CTRL) == (false))) && (((VENT_PACE_CTRL ) == (true)))]
  (junction 1073745818) -> (junction 1073745826) [order 2]
  (junction 1073745820) -> (junction 1073745822) : {
      | reqtable_postcondition((PACE_GND_CTRL == true) && (((ATR_GND_CTRL ) == (false))) && (((VENT_GND_CTRL ) == (true))) && (((FRONT_END_CTRL ) == (true))) && (((Z_ATR_CTRL) == (false))) && (((Z_VENT_CTRL) == (false))), 'R:6');
      |
      |
      | }
  (junction 1073745822) -> (junction 1073745824) : {
      | }
  (junction 1073745824) -> (junction 1073745826)
  (junction 1073745826) -> (junction 1073745828)
  (junction 1073745828) -> (junction 1073745830) : {
      | % END_R_16
      | }
  data: MODE input; VENT_PACE_CTRL input; PACE_CHARGE_CTRL input; FRONT_END_CTRL input; VENT_GND_CTRL input; PACE_GND_CTRL input; ATR_GND_CTRL input; ATR_PACE_CTRL input; Z_VENT_CTRL input; Z_ATR_CTRL input

== stateflow chart Improved_Final_Model/COM_IN ==
  state SET_PARAM
    entry:
    ATR_AMP = cast(rxdata(3),'uint8');
    ATR_PW = cast(rxdata(4),'uint8');
    Mode =cast(rxdata(5),'uint8');
    VENT_AMP = cast(rxdata(6),'uint8');
    VENT_PW = cast(rxdata(7),'uint8');
    ARP = cast(rxdata(8),'uint8');
    VRP = cast(rxdata(9),'uint8');
    LRL = cast(rxdata(10),'uint8');
    Activity_Threshold =cast(rxdata(11),'uint8');
    Response_Factor =cast(rxdata(12),'uint8');
    Recovery_Time = cast(rxdata(13),'uint8');
    Max_Sensor_Rate =cast(rxdata(14),'uint8');
    Reaction_Time = cast(rxdata(15),'uint8');
  state INITIAL
    entry:
    ATR_AMP = cast(5,'uint8');
    ATR_PW = cast(10,'uint8');
    Mode =cast(2,'uint8');
    VENT_AMP =cast(5,'uint8');
    VENT_PW = cast(10,'uint8');
    ARP =cast(250,'uint8');
    VRP =cast(250,'uint8');
    LRL = cast(60,'uint8');
    Activity_Threshold =cast(5,'uint8');
    Response_Factor = cast(5,'uint8');
    Recovery_Time = cast(5,'uint8');
    Max_Sensor_Rate =cast(5,'uint8');
    Reaction_Time = cast(5,'uint8');
  state STANDBY
  state ECHO_PARAM
    entry:
    send_Test();
  (default) -> INITIAL
  SET_PARAM -> STANDBY
  (junction 15) -> SET_PARAM [order 1] : [rxdata(2)==hex2dec('55')]
  (junction 14) -> STANDBY [order 2]
  INITIAL -> STANDBY
  STANDBY -> (junction 14) : [status==0]
  (junction 14) -> (junction 15) [order 1] : [rxdata(1)==hex2dec('16')]
  (junction 15) -> ECHO_PARAM [order 2] : [rxdata(2)==hex2dec('22')]
  ECHO_PARAM -> STANDBY
  data: rxdata input uint8; status input uint8; ATR_PW output; ATR_AMP output; Mode output; VENT_AMP output; VENT_PW output; ARP output; VRP output; LRL output; Activity_Threshold output; Response_Factor output; Recovery_Time output; Max_Sensor_Rate output; Reaction_Time output

== stateflow chart Improved_Final_Model/Input Parameter Requirements1 ==
  (default) -> (junction 1073742081)
  (junction 1073742081) -> (junction 1073742082) : {
      | % SF_REQ_REV_07
      | }
  (junction 1073742082) -> (junction 1073742084) : {
      | % HEADER_ASSIGNMENTS
      |
      | }
  (junction 1073742084) -> (junction 1073742086) : {
      | % START_A_4
      | }
  (junction 1073742086) -> (junction 1073742088) : {
      | }
  (junction 1073742088) -> (junction 1073742090)
  (junction 1073742090) -> (junction 1073742092) : {
      | }
  (junction 1073742092) -> (junction 1073742094) : {
      | % END_A_4
      | }
  (junction 1073742094) -> (junction 1073742096) : {
      | % START_R_1
      | }
  (junction 1073742096) -> (junction 1073742098) : {
      | }
  (junction 1073742098) -> (junction 1073742100) : {
      | reqtable_postcondition((((p_aPaceAmp) == (0 || [0.112, 5.6]))) && (((p_vPaceAmp) == (0 || [0.112, 5.6]))) && (((p_aPaceWidth) >= (1) && (p_aPaceWidth) <= (31))) && (((p_vPaceWidth) >= (1) && (p_vPaceWidth) <= (31))) && (((p_aSensitivity) >= (0) && (p_aSensitivity) <= (5))) && (((p_vSensitivity) >= (0) && (p_vSensitivity) <= (5))) && ([150,500] && p_aPaceWidth < (p_ARP)< p_lowrateInterval) && ([150,500] && p_vPaceWidth < (p_VRP) < p_lowrateInterval) && (((p_lowrateInterval ) >= (343) && (p_lowrateInterval ) <= (2000))) && (((p_pacingMode ) == (1)) || ((p_pacingMode ) == (2)) || ((p_pacingMode ) == (3)) || ((p_pacingMode ) == (4)) || ((p_pacingMode ) == (5))), 'R:1');
      |
      |
      | }
  (junction 1073742100) -> (junction 1073742102) : {
      | }
  (junction 1073742102) -> (junction 1073742104) : {
      | % END_R_1
      | }
  data: p_aPaceWidth input; p_vPaceWidth input; p_vSensitivity input; p_aSensitivity input; p_vPaceAmp input; p_pacingMode input; p_lowrateInterval input; p_aPaceAmp input; p_VRP input; p_ARP input

== stateflow chart Improved_Final_Model/Subsystem2/Chart ==
  state S2FAIL1
    entry:
    AdaptedRate = AdaptedRate - step_down;
  state S4
    entry:
    AdaptedRate = AdaptedRate + step_up;
  state S3
    entry:
    AdaptedRate = TargetRate;
  state Start1
    entry:
    AdaptedRate = LOWER_RATE_LIMIT;
  state S_FAILSAFE1
    entry:
    AdaptedRate = AdaptedRate - step_up;
  S_FAILSAFE1 -> S2FAIL1 [order 2] : [ after(1000,msec)]
  S2FAIL1 -> Start1 [order 1] : [AdaptedRate <= LOWER_RATE_LIMIT]
  S2FAIL1 -> S4 [order 3] : [AccelerateYorN == 1]
  S2FAIL1 -> S2FAIL1 [order 2] : after(1000, msec)[AdaptedRate >= LOWER_RATE_LIMIT]
  S3 -> S2FAIL1 [order 2] : [AccelerateYorN == 0]
  (default) -> Start1 : {step_up = ceil((TargetRate - LOWER_RATE_LIMIT) / ReactionTime),
      | step_down = ceil((TargetRate - LOWER_RATE_LIMIT)  / RecoveryTime)}
  S4 -> S4 [order 1] : after(1000,msec)[AdaptedRate <= TargetRate]
  S4 -> S3 [order 3] : [AdaptedRate >= TargetRate]
  Start1 -> S4 [order 1] : [AccelerateYorN == 1]
  Start1 -> Start1 [order 2] : [AccelerateYorN == 0]
  S3 -> S3 [order 1] : [AccelerateYorN == 1]
  S4 -> S_FAILSAFE1 [order 2] : [AccelerateYorN == 0]
  S_FAILSAFE1 -> S4 [order 1] : [AccelerateYorN == 1]
  data: step_down local; step_up local; LOWER_RATE_LIMIT input; AccelerateYorN input; ReactionTime input; RecoveryTime input; AdaptedRate output; TargetRate input
